simulink model "linecode"  (R2015a)
settings: Solver=ode45  StartTime=0.0  StopTime=10.0  RelTol=1e-3
undefined symbols (not defined in the file or in its folder): get
libraries: simulink_extras x2, commrandsrc2 x1, dspxfrm3 x1, commutil2 x1, dspsnks4 x1
settings Model: Creator=Sonu Sharma  LastModifiedBy=Sonu Sharma

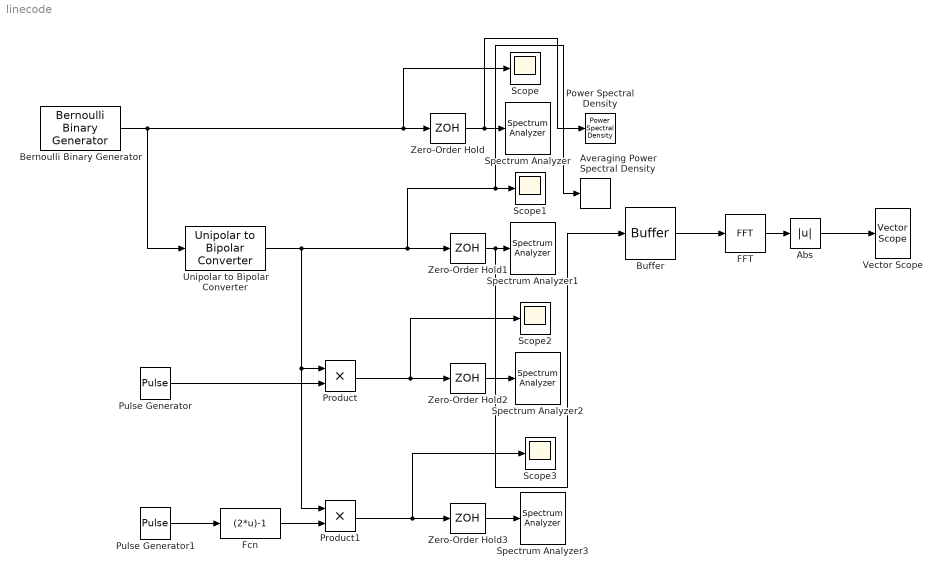
== system linecode ==
  Abs : Abs
  Averaging Power Spectral Density : simulink_extras/Additional Sinks/Averaging Power Spectral Density  npts=128  fftpts=512  HowOften=64  sampleT=0.1
  Bernoulli Binary Generator : commrandsrc2/Bernoulli Binary Generator  P=0.5  seed=61  Ts=1  frameBased=off  sampPerFrame=1  orient=off  outDataType=double
  Buffer : Buffer  N=128  TreatMby1Signals=One channel
  FFT : dspxfrm3/FFT  CompMethod=Table lookup  TableOpt=NEW  TableOptActive=Speed  BitRevOrder=off  InheritFFTLength=off  FFTLength=512  WrapInput=on  RowConvenienceOn=on  FFTImplementation=Auto  SkipNorm=off  firstCoeffDataTypeStr=Inherit: Same word length as input  firstCoeffLastDataTypeStr=Inherit: Same word length as input  outputMin=[]  outputMax=[]  roundingMode=Floor  overflowMode=off
  Fcn : Fcn  Expr=(2*u)-1
  Power Spectral Density : simulink_extras/Additional Sinks/Power Spectral Density  npts=128  fftpts=512  HowOften=64  sampleT=0.1
  Product : Product
  Product1 : Product
  Pulse Generator : DiscretePulseGenerator  PulseType=Time based  Period=1  PulseWidth=50
  Pulse Generator1 : DiscretePulseGenerator  PulseType=Time based  Period=1  PulseWidth=50
  Scope{,1..3} (4 alike) : Scope
      Scope2 settings: SaveName=ScopeData2
      Scope3 settings: SaveName=ScopeData3
  Spectrum Analyzer{,1..3} (4 alike) : SpectrumAnalyzer
  Unipolar to Bipolar Converter : commutil2/Unipolar to Bipolar Converter  M=2  polarity=Positive  dataType=Inherit via internal rule
  Vector Scope : dspsnks4/Vector Scope  ScopeProperties=on  Domain=Time  HorizSpan=1  DisplayProperties=off  AxisGrid=on  Memory=off  FrameNumber=on  AxisLegend=off  AxisZoom=off  OpenScopeAtSimStart=on  OpenScopeImmediately=off  FigPos=get(0,'defaultfigureposition')  AxisProperties=off  XUnits=Hertz  XRange=[0...Fs/2]  InheritXIncr=on  XIncr=1  XLabel=Time  XLimit=Auto  XMin=0  XMax=1  XStart=0  YUnits=dB  YLabel=Amplitude  LineProperties=off  XAxisParamsVer=6.9
      settings: YMin=-10  YMax=10
  Zero-Order Hold{,1..3} (4 alike) : ZeroOrderHold  SampleTime=1/32
  wires:
  Pulse Generator/1 -> Product/2
  Bernoulli Binary Generator/1 -> Scope/1, Zero-Order Hold/1, Unipolar to Bipolar Converter/1
  Zero-Order Hold2/1 -> Spectrum Analyzer2/1
  Product/1 -> Zero-Order Hold2/1, Scope2/1
  Pulse Generator1/1 -> Fcn/1
  Zero-Order Hold3/1 -> Spectrum Analyzer3/1
  Product1/1 -> Scope3/1, Zero-Order Hold3/1
  Fcn/1 -> Product1/2
  Unipolar to Bipolar Converter/1 -> Product1/1, Product/1, Zero-Order Hold1/1, Averaging Power Spectral Density/1, Scope1/1
  Buffer/1 -> FFT/1
  Zero-Order Hold1/1 -> Buffer/1, Spectrum Analyzer1/1
  FFT/1 -> Abs/1
  Abs/1 -> Vector Scope/1
  Zero-Order Hold/1 -> Power Spectral Density/1, Spectrum Analyzer/1
